simulink model "test_ode"  (R2018b)
settings: Solver=FixedStepDiscrete  StartTime=0.0  StopTime=10.0  RelTol=1e-3
libraries: powerlib x6
settings Model: Creator=yg934  LastModifiedBy=yg934

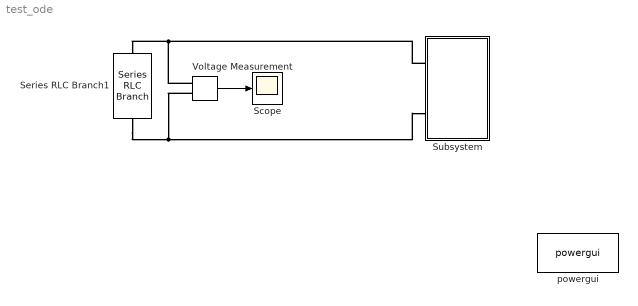
== system test_ode ==
  Scope : Scope
  Series RLC Branch1 : powerlib/Elements/Series RLC Branch  LConnTagsString=__new0  RConnTagsString=__new0  BranchType=C  Resistance=1  Inductance=1e-3  SetiL0=off  InitialCurrent=0  Capacitance=1e-3  Setx0=off  InitialVoltage=0  Measurements=None
  Subsystem : Subsystem  mask{Inductance=1e-3, SampleTime=5e-5}
      mask prompts: SampleTime "Sample Time"
      mask init:
      | obj = SimplexPS.Class.Inductor('Para',Inductance,'Ts',SampleTime);
      | Rv = obj.GetVirtualResistor(obj);
      | blk = [gcb '/Rv'];
      | set_param(blk,'Resistance',num2str(Rv));
  Voltage Measurement : powerlib/Measurements/Voltage Measurement  PhasorSimulation=off  OutputType=Complex  PSBequivalent=0
  powergui : powerlib/powergui  Priority=1  SimulationMode=Discrete  SampleTime=50e-6  frequency=60  Iterations=50  frequencyindice=0  Pbase=100e6  ErrMax=1e-4  UnitsV=kV  UnitsW=MW  buscounter=0  FunctionMessages=off  echomessages=off  EnableUseOfTLC=off  CurrentSourceSwitches=off  DisableSnubberDevices=off  DisableRonSwitches=off  DisableVfSwitches=off  DisplayEquations=off  SolverType=Tustin  Interpol=off  ExternalGateDelay=off  methode=off  Ts=100  x0status=blocks  SPID=on  SwTol=0  HookPort=off  RestoreLinks=warning  ResistiveCurrentMeasurement=off  Frange=[0:2:500]  Ylog=off  Xlog=on  ShowGrid=off  save=off  variable=ZData  structure=0  ZoomFFT=off  StartTime=0.0  cycles=1  DisplayStyle=1  fundamental=60  FreqAxis=off  MaxFrequency=1000  frequencyindicesteady=1  RmsSteady=1  display=off
  wires:
  Voltage Measurement/1 -> Scope/1
  connections:
  Subsystem/LConn1 -- Voltage Measurement/LConn1 -- Series RLC Branch1/LConn1
  Series RLC Branch1/RConn1 -- Voltage Measurement/LConn2 -- Subsystem/LConn2

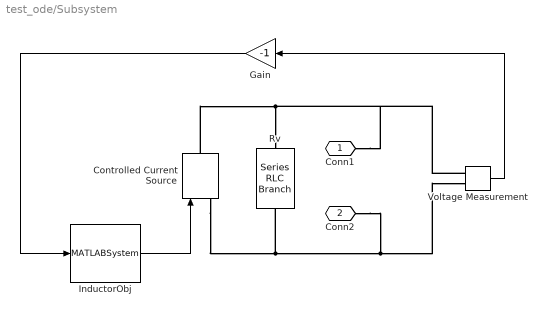
== system test_ode/Subsystem ==
  Controlled Current Source : powerlib/Electrical Sources/Controlled Current Source  Initialize=on  Source_Type=AC  Amplitude=0  Phase=0  Frequency=0  Measurements=None
  Gain : Gain  Gain=-1
  InductorObj : MATLABSystem  System=SimplexPS.Class.Inductor  Ts=SampleTime  Para=Inductance  PowerFlow=[]  x0=1  DiscreMethod=2  LinearizationTimes=1  VoidJacobStates=[]  VoidFeedthrough=[]  DiscreDampingFlag=1  ElecPortIOs=[1]  EquiInitial=0  DeviceType=[]  DirectFeedthrough=0  SimulateUsing=Code generation
      mask Type: SimplexPS.Class.Inductor
      mask Display:
      | disp('Inductor');
      | port_label('input',1,'u');
      | port_label('output',1,'y');
  Rv : powerlib/Elements/Series RLC Branch  LConnTagsString=__new0  RConnTagsString=__new0  BranchType=R  Resistance=40  Inductance=1e-3  SetiL0=off  InitialCurrent=0  Capacitance=1e-6  Setx0=off  InitialVoltage=0  Measurements=None
  Voltage Measurement : powerlib/Measurements/Voltage Measurement  PhasorSimulation=off  OutputType=Complex  PSBequivalent=0
  Conn1 : PMIOPort  Side=Left
  Conn2 : PMIOPort  Port=2  Side=Left
  wires:
  InductorObj/1 -> Controlled Current Source/1
  Gain/1 -> InductorObj/1
  Voltage Measurement/1 -> Gain/1
  connections:
  Controlled Current Source/RConn1 -- Conn1/RConn1 -- Voltage Measurement/LConn1 -- Rv/LConn1
  Controlled Current Source/LConn1 -- Rv/RConn1 -- Conn2/RConn1 -- Voltage Measurement/LConn2
